simulink model "BANSHEE"  (Simulink 8.7)
settings: Solver=ode1  StartTime=0.0  StopTime=inf  FixedStep=Ts  MaxStep=1e-3  RelTol=1e-3
PostLoadFcn:
  | BANSHEE_init;
InitFcn:
  | BANSHEE_init;
values from neighbouring files (symbols this model uses):
  Ts = 100E-6    (= 0.0001)    [BANSHEE_init.m]
undefined symbols (not defined in the file or in its folder): Acid, Banshee_HWCtrl_IOs, Banshee_SEL751_Woodward_lib, DMS_slave_lib, DMSCommands, F1, F2, F3, fdesignblkfcn, Feeder1_lib, Feeder2_lib, Feeder3_lib, gcbh, generic_ethernet_cb, Lead, Left, relay_housing_lib, SM_UtilityService, SS_F1_RELAY_HOUSING, SS_F2_RELAY_HOUSING, SS_F3_RELAY_HOUSING, SS_Feeder1, SS_Feeder2, SS_Feeder3, SUBSTATION, TestSeq_slave_lib, TestSequenceCommands, type, utility_service_lib, V
libraries: powerlib x108, cables_lib x61, breaker_lib x53, rtio_generic_modbus x50, relay_modbus_lib x45, rtio_opalrt_op5142ex1 x37, transformer_lib x29, rteventslib x28, Load_lib x25, simulink x24, rtlab x20, ssn_lib x19
(part 7 of 9)

== system BANSHEE/SS_PV_BESS/EPC/LCL Filter 200kW1 ==
  note: High Resistor:
      | 10e6 ohms
      | Numerical Stability
  note: Create a three wire version that removes the Inv 4 port and 4 nuetral.
      | There is a reistor in parallel with the capacitor for the discharge voltage at shutoff.
  Bleed_R1 : powerlib/Elements/Series RLC Branch  LConnTagsString=__new0  RConnTagsString=__new0  BranchType=R  Resistance=filter_cap_bleed_res  Inductance=1e-3  SetiL0=off  InitialCurrent=0  Capacitance=filter_cap  Setx0=on  InitialVoltage=0  Measurements=None
  Bleed_R2 : powerlib/Elements/Series RLC Branch  LConnTagsString=__new0  RConnTagsString=__new0  BranchType=R  Resistance=filter_cap_bleed_res  Inductance=1e-3  SetiL0=off  InitialCurrent=0  Capacitance=filter_cap  Setx0=on  InitialVoltage=0  Measurements=None
  Bleed_R3 : powerlib/Elements/Series RLC Branch  LConnTagsString=__new0  RConnTagsString=__new0  BranchType=R  Resistance=filter_cap_bleed_res  Inductance=1e-3  SetiL0=off  InitialCurrent=0  Capacitance=filter_cap  Setx0=on  InitialVoltage=0  Measurements=None
  Capacitor_L1 : powerlib/Elements/Series RLC Branch  LConnTagsString=__new0  RConnTagsString=__new0  BranchType=RC  Resistance=filter_cap_res  Inductance=1e-3  SetiL0=off  InitialCurrent=0  Capacitance=filter_cap  Setx0=on  InitialVoltage=0  Measurements=None
  Capacitor_L2 : powerlib/Elements/Series RLC Branch  LConnTagsString=__new0  RConnTagsString=__new0  BranchType=RC  Resistance=filter_cap_res  Inductance=1e-3  SetiL0=off  InitialCurrent=0  Capacitance=filter_cap  Setx0=on  InitialVoltage=0  Measurements=None
  Capacitor_L3 : powerlib/Elements/Series RLC Branch  LConnTagsString=__new0  RConnTagsString=__new0  BranchType=RC  Resistance=filter_cap_res  Inductance=1e-3  SetiL0=off  InitialCurrent=0  Capacitance=filter_cap  Setx0=on  InitialVoltage=0  Measurements=None
  Inductor_Inv1 : powerlib/Elements/Series RLC Branch  LConnTagsString=__new0  RConnTagsString=__new0  BranchType=RL  Resistance=filter_inv_res  Inductance=filter_inv_ind  SetiL0=off  InitialCurrent=0  Capacitance=1e-6  Setx0=off  InitialVoltage=0  Measurements=None
  Inductor_Inv2 : powerlib/Elements/Series RLC Branch  LConnTagsString=__new0  RConnTagsString=__new0  BranchType=RL  Resistance=filter_inv_res  Inductance=filter_inv_ind  SetiL0=off  InitialCurrent=0  Capacitance=1e-6  Setx0=off  InitialVoltage=0  Measurements=None
  Inductor_Inv3 : powerlib/Elements/Series RLC Branch  LConnTagsString=__new0  RConnTagsString=__new0  BranchType=RL  Resistance=filter_inv_res  Inductance=filter_inv_ind  SetiL0=off  InitialCurrent=0  Capacitance=1e-6  Setx0=off  InitialVoltage=0  Measurements=None
  Inductor_Inv4 : powerlib/Elements/Series RLC Branch  LConnTagsString=__new0  RConnTagsString=__new0  BranchType=L  Resistance=1  Inductance=filter_inv_ind  SetiL0=off  InitialCurrent=0  Capacitance=1e-6  Setx0=off  InitialVoltage=0  Measurements=None
  Inductor_L1 : powerlib/Elements/Series RLC Branch  LConnTagsString=__new0  RConnTagsString=__new0  BranchType=RL  Resistance=filter_line_res  Inductance=filter_line_ind  SetiL0=off  InitialCurrent=0  Capacitance=1e-6  Setx0=off  InitialVoltage=0  Measurements=None
  Inductor_L2 : powerlib/Elements/Series RLC Branch  LConnTagsString=__new0  RConnTagsString=__new0  BranchType=RL  Resistance=filter_line_res  Inductance=filter_line_ind  SetiL0=off  InitialCurrent=0  Capacitance=1e-6  Setx0=off  InitialVoltage=0  Measurements=None
  Inductor_L3 : powerlib/Elements/Series RLC Branch  LConnTagsString=__new0  RConnTagsString=__new0  BranchType=RL  Resistance=filter_line_res  Inductance=filter_line_ind  SetiL0=off  InitialCurrent=0  Capacitance=1e-6  Setx0=off  InitialVoltage=0  Measurements=None
  Three-Phase Series RLC Branch : powerlib/Elements/Three-Phase Series RLC Branch  LConnTagsString=A|B|C  RConnTagsString=A|B|C  BranchType=R  Resistance=1e6  Inductance=1e-3  Capacitance=1e-6  Measurements=None
  A : PMIOPort  Port=1  Side=Left
  B : PMIOPort  Port=2  Side=Left
  C : PMIOPort  Port=3  Side=Left
  N : PMIOPort  Port=4  Side=Left
  Inv_1 : PMIOPort  Port=5  Side=Right  mask{filter_line_ind=[], filter_cap=0, filter_inv_ind=0}
      mask prompts: filter_line_ind "Line Filter Inductor (H)"; filter_cap "Filter Capacitor (F)"; filter_inv_ind "Inverter Filter Inductor (H)"
  Inv_2 : PMIOPort  Port=6  Side=Right
  Inv_3 : PMIOPort  Port=7  Side=Right
  Inv_4 : PMIOPort  Port=8  Side=Right
  connections:
  Inductor_L1/RConn1 -- Inductor_Inv1/LConn1 -- Capacitor_L1/LConn1 -- Bleed_R1/LConn1
  Inv_1/RConn1 -- Inductor_Inv1/RConn1
  A/RConn1 -- Inductor_L1/LConn1
  Inductor_L2/RConn1 -- Inductor_Inv2/LConn1 -- Capacitor_L2/LConn1 -- Bleed_R2/LConn1
  Inv_2/RConn1 -- Inductor_Inv2/RConn1
  B/RConn1 -- Inductor_L2/LConn1
  Inductor_L3/RConn1 -- Inductor_Inv3/LConn1 -- Capacitor_L3/LConn1 -- Bleed_R3/LConn1
  Inv_3/RConn1 -- Inductor_Inv3/RConn1
  C/RConn1 -- Inductor_L3/LConn1
  N/RConn1 -- Capacitor_L1/RConn1 -- Bleed_R1/RConn1 -- Capacitor_L2/RConn1 -- Bleed_R2/RConn1 -- Capacitor_L3/RConn1 -- Bleed_R3/RConn1 -- Inductor_Inv4/LConn1
  Inv_4/RConn1 -- Inductor_Inv4/RConn1

== system BANSHEE/SS_PV_BESS/EPC/LCL Filter 200kW2 ==
  note: High Resistor:
      | 10e6 ohms
      | Numerical Stability
  note: Create a three wire version that removes the Inv 4 port and 4 nuetral.
      | There is a reistor in parallel with the capacitor for the discharge voltage at shutoff.
  Bleed_R1 : powerlib/Elements/Series RLC Branch  LConnTagsString=__new0  RConnTagsString=__new0  BranchType=R  Resistance=filter_cap_bleed_res  Inductance=1e-3  SetiL0=off  InitialCurrent=0  Capacitance=filter_cap  Setx0=on  InitialVoltage=0  Measurements=None
  Bleed_R2 : powerlib/Elements/Series RLC Branch  LConnTagsString=__new0  RConnTagsString=__new0  BranchType=R  Resistance=filter_cap_bleed_res  Inductance=1e-3  SetiL0=off  InitialCurrent=0  Capacitance=filter_cap  Setx0=on  InitialVoltage=0  Measurements=None
  Bleed_R3 : powerlib/Elements/Series RLC Branch  LConnTagsString=__new0  RConnTagsString=__new0  BranchType=R  Resistance=filter_cap_bleed_res  Inductance=1e-3  SetiL0=off  InitialCurrent=0  Capacitance=filter_cap  Setx0=on  InitialVoltage=0  Measurements=None
  Capacitor_L1 : powerlib/Elements/Series RLC Branch  LConnTagsString=__new0  RConnTagsString=__new0  BranchType=RC  Resistance=filter_cap_res  Inductance=1e-3  SetiL0=off  InitialCurrent=0  Capacitance=filter_cap  Setx0=on  InitialVoltage=0  Measurements=None
  Capacitor_L2 : powerlib/Elements/Series RLC Branch  LConnTagsString=__new0  RConnTagsString=__new0  BranchType=RC  Resistance=filter_cap_res  Inductance=1e-3  SetiL0=off  InitialCurrent=0  Capacitance=filter_cap  Setx0=on  InitialVoltage=0  Measurements=None
  Capacitor_L3 : powerlib/Elements/Series RLC Branch  LConnTagsString=__new0  RConnTagsString=__new0  BranchType=RC  Resistance=filter_cap_res  Inductance=1e-3  SetiL0=off  InitialCurrent=0  Capacitance=filter_cap  Setx0=on  InitialVoltage=0  Measurements=None
  Inductor_Inv1 : powerlib/Elements/Series RLC Branch  LConnTagsString=__new0  RConnTagsString=__new0  BranchType=RL  Resistance=filter_inv_res  Inductance=filter_inv_ind  SetiL0=off  InitialCurrent=0  Capacitance=1e-6  Setx0=off  InitialVoltage=0  Measurements=None
  Inductor_Inv2 : powerlib/Elements/Series RLC Branch  LConnTagsString=__new0  RConnTagsString=__new0  BranchType=RL  Resistance=filter_inv_res  Inductance=filter_inv_ind  SetiL0=off  InitialCurrent=0  Capacitance=1e-6  Setx0=off  InitialVoltage=0  Measurements=None
  Inductor_Inv3 : powerlib/Elements/Series RLC Branch  LConnTagsString=__new0  RConnTagsString=__new0  BranchType=RL  Resistance=filter_inv_res  Inductance=filter_inv_ind  SetiL0=off  InitialCurrent=0  Capacitance=1e-6  Setx0=off  InitialVoltage=0  Measurements=None
  Inductor_Inv4 : powerlib/Elements/Series RLC Branch  LConnTagsString=__new0  RConnTagsString=__new0  BranchType=L  Resistance=1  Inductance=filter_inv_ind  SetiL0=off  InitialCurrent=0  Capacitance=1e-6  Setx0=off  InitialVoltage=0  Measurements=None
  Inductor_L1 : powerlib/Elements/Series RLC Branch  LConnTagsString=__new0  RConnTagsString=__new0  BranchType=RL  Resistance=filter_line_res  Inductance=filter_line_ind  SetiL0=off  InitialCurrent=0  Capacitance=1e-6  Setx0=off  InitialVoltage=0  Measurements=None
  Inductor_L2 : powerlib/Elements/Series RLC Branch  LConnTagsString=__new0  RConnTagsString=__new0  BranchType=RL  Resistance=filter_line_res  Inductance=filter_line_ind  SetiL0=off  InitialCurrent=0  Capacitance=1e-6  Setx0=off  InitialVoltage=0  Measurements=None
  Inductor_L3 : powerlib/Elements/Series RLC Branch  LConnTagsString=__new0  RConnTagsString=__new0  BranchType=RL  Resistance=filter_line_res  Inductance=filter_line_ind  SetiL0=off  InitialCurrent=0  Capacitance=1e-6  Setx0=off  InitialVoltage=0  Measurements=None
  Three-Phase Series RLC Branch : powerlib/Elements/Three-Phase Series RLC Branch  LConnTagsString=A|B|C  RConnTagsString=A|B|C  BranchType=R  Resistance=1e6  Inductance=1e-3  Capacitance=1e-6  Measurements=None
  A : PMIOPort  Port=1  Side=Left
  B : PMIOPort  Port=2  Side=Left
  C : PMIOPort  Port=3  Side=Left
  N : PMIOPort  Port=4  Side=Left
  Inv_1 : PMIOPort  Port=5  Side=Right  mask{filter_line_ind=[], filter_cap=0, filter_inv_ind=0}
      mask prompts: filter_line_ind "Line Filter Inductor (H)"; filter_cap "Filter Capacitor (F)"; filter_inv_ind "Inverter Filter Inductor (H)"
  Inv_2 : PMIOPort  Port=6  Side=Right
  Inv_3 : PMIOPort  Port=7  Side=Right
  Inv_4 : PMIOPort  Port=8  Side=Right
  connections:
  Inductor_L1/RConn1 -- Inductor_Inv1/LConn1 -- Capacitor_L1/LConn1 -- Bleed_R1/LConn1
  Inv_1/RConn1 -- Inductor_Inv1/RConn1
  A/RConn1 -- Inductor_L1/LConn1
  Inductor_L2/RConn1 -- Inductor_Inv2/LConn1 -- Capacitor_L2/LConn1 -- Bleed_R2/LConn1
  Inv_2/RConn1 -- Inductor_Inv2/RConn1
  B/RConn1 -- Inductor_L2/LConn1
  Inductor_L3/RConn1 -- Inductor_Inv3/LConn1 -- Capacitor_L3/LConn1 -- Bleed_R3/LConn1
  Inv_3/RConn1 -- Inductor_Inv3/RConn1
  C/RConn1 -- Inductor_L3/LConn1
  N/RConn1 -- Capacitor_L1/RConn1 -- Bleed_R1/RConn1 -- Capacitor_L2/RConn1 -- Bleed_R2/RConn1 -- Capacitor_L3/RConn1 -- Bleed_R3/RConn1 -- Inductor_Inv4/LConn1
  Inv_4/RConn1 -- Inductor_Inv4/RConn1

== system BANSHEE/SC_ctrl/EPC Inverter/16TSDIn/16 TSDOut GR3/Din/Dout ch16-23 ==
  Bus Creator3 : BusCreator  Inputs=8
  times17 : Constant  Value=[0.05 0.15 0.25 0.35]
  times18 : Constant  Value=[0.1 0.2 0.3 0.4]
  times19 : Constant  Value=[0.15 0.25 0.35 0.45]
  times20 : Constant  Value=[0.2 0.3 0.4 0.5]
  times21 : Constant  Value=[0.25 0.35 0.45 0.55]
  times22 : Constant  Value=[0.3 0.4 0.5 0.6]
  times23 : Constant  Value=[0.3 0.4 0.5 0.6]
  times24 : Constant  Value=[0 0.1 0.2 0.3]
  Out1 : Outport
  wires:
  times24/1 -> Bus Creator3/1  "times17"
  times17/1 -> Bus Creator3/2  "times18"
  times18/1 -> Bus Creator3/3  "times19"
  times19/1 -> Bus Creator3/4  "times20"
  times20/1 -> Bus Creator3/5  "times21"
  times21/1 -> Bus Creator3/6  "times22"
  times22/1 -> Bus Creator3/7  "times23"
  times23/1 -> Bus Creator3/8  "times24"
  Bus Creator3/1 -> Out1/1

== system BANSHEE/SC_ctrl/EPC Inverter/16TSDIn/16 TSDOut GR3/Din/Dout ch24-31 ==
  Bus Creator4 : BusCreator  Inputs=8
  times25 : Constant  Value=[0.05 0.15 0.25 0.35]
  times26 : Constant  Value=[0.1 0.2 0.3 0.4]
  times27 : Constant  Value=[0.15 0.25 0.35 0.45]
  times28 : Constant  Value=[0.2 0.3 0.4 0.5]
  times29 : Constant  Value=[0.25 0.35 0.45 0.55]
  times30 : Constant  Value=[0.3 0.4 0.5 0.6]
  times31 : Constant  Value=[0.3 0.4 0.5 0.6]
  times32 : Constant  Value=[0 0.1 0.2 0.3]
  Out1 : Outport
  wires:
  times32/1 -> Bus Creator4/1  "times25"
  times25/1 -> Bus Creator4/2  "times26"
  times26/1 -> Bus Creator4/3  "times27"
  times27/1 -> Bus Creator4/4  "times28"
  times28/1 -> Bus Creator4/5  "times29"
  times29/1 -> Bus Creator4/6  "times30"
  times30/1 -> Bus Creator4/7  "times31"
  times31/1 -> Bus Creator4/8  "times32"
  Bus Creator4/1 -> Out1/1

== system BANSHEE/SC_ctrl/EPC Inverter/16TSDIn/16 TSDOut GR3/Dout state ctrl ==
  Bus Creator : BusCreator  Inputs=2
  Dout_CH16_CH23 : Subsystem
  Dout_CH24_CH31 : Subsystem
  Event State OUT : Outport
  wires:
  Bus Creator/1 -> Event State OUT/1
  Dout_CH16_CH23/1(Dout_CH8_CH15) -> Bus Creator/1  "CH16-23"
  Dout_CH24_CH31/1(Dout_CH8_CH15) -> Bus Creator/2  "CH24-31"

== system BANSHEE/SM_UtilityService/Banshee_HWCtrl_IOs/SEL751_DigitalAnalog_IO_OpBlocks/F1 ==
  Substation : Inport
  Feeder : Inport  Port=2
  DTT : Inport  Port=3
  TS_SQ : Inport  Port=4
  Logical Operator : Logic  AllPortsSameDT=off  OutDataTypeStr=boolean
  Logical Operator1 : Logic  Operator=OR  Inputs=3  AllPortsSameDT=off  OutDataTypeStr=boolean
  Logical Operator2 : Logic  Operator=OR  AllPortsSameDT=off  OutDataTypeStr=boolean
  Logical Operator3 : Logic  Operator=NOT  AllPortsSameDT=off  OutDataTypeStr=boolean
  Logical Operator5 : Logic  Operator=NOT  AllPortsSameDT=off  OutDataTypeStr=boolean
  trip : Outport
  wires:
  DTT/1 -> Logical Operator2/1
  Feeder/1 -> Logical Operator5/1
  Logical Operator5/1 -> Logical Operator1/2
  Substation/1 -> Logical Operator3/1
  Logical Operator3/1 -> Logical Operator1/1
  Logical Operator1/1 -> Logical Operator/1
  Logical Operator/1 -> trip/1
  Logical Operator2/1 -> Logical Operator/2
  TS_SQ/1 -> Logical Operator1/3, Logical Operator2/2

== system BANSHEE/SM_UtilityService/Banshee_HWCtrl_IOs/SEL751_DigitalAnalog_IO_OpBlocks/F2 ==
  Substation : Inport
  Feeder : Inport  Port=2
  DTT : Inport  Port=3
  TS_SQ : Inport  Port=4
  Logical Operator : Logic  AllPortsSameDT=off  OutDataTypeStr=boolean
  Logical Operator1 : Logic  Operator=OR  Inputs=3  AllPortsSameDT=off  OutDataTypeStr=boolean
  Logical Operator2 : Logic  Operator=OR  AllPortsSameDT=off  OutDataTypeStr=boolean
  Logical Operator3 : Logic  Operator=NOT  AllPortsSameDT=off  OutDataTypeStr=boolean
  Logical Operator5 : Logic  Operator=NOT  AllPortsSameDT=off  OutDataTypeStr=boolean
  trip : Outport
  wires:
  DTT/1 -> Logical Operator2/1
  Feeder/1 -> Logical Operator5/1
  Logical Operator5/1 -> Logical Operator1/2
  Substation/1 -> Logical Operator3/1
  Logical Operator3/1 -> Logical Operator1/1
  Logical Operator1/1 -> Logical Operator/1
  Logical Operator/1 -> trip/1
  Logical Operator2/1 -> Logical Operator/2
  TS_SQ/1 -> Logical Operator1/3, Logical Operator2/2

== system BANSHEE/SM_UtilityService/Banshee_HWCtrl_IOs/SEL751_DigitalAnalog_IO_OpBlocks/F3 ==
  Substation : Inport
  Feeder : Inport  Port=2
  DTT : Inport  Port=3
  TS_SQ : Inport  Port=4
  Logical Operator : Logic  AllPortsSameDT=off  OutDataTypeStr=boolean
  Logical Operator1 : Logic  Operator=OR  Inputs=3  AllPortsSameDT=off  OutDataTypeStr=boolean
  Logical Operator2 : Logic  Operator=OR  AllPortsSameDT=off  OutDataTypeStr=boolean
  Logical Operator3 : Logic  Operator=NOT  AllPortsSameDT=off  OutDataTypeStr=boolean
  Logical Operator5 : Logic  Operator=NOT  AllPortsSameDT=off  OutDataTypeStr=boolean
  trip : Outport
  wires:
  DTT/1 -> Logical Operator2/1
  Feeder/1 -> Logical Operator5/1
  Logical Operator5/1 -> Logical Operator1/2
  Substation/1 -> Logical Operator3/1
  Logical Operator3/1 -> Logical Operator1/1
  Logical Operator1/1 -> Logical Operator/1
  Logical Operator/1 -> trip/1
  Logical Operator2/1 -> Logical Operator/2
  TS_SQ/1 -> Logical Operator1/3, Logical Operator2/2

== system BANSHEE/SM_UtilityService/Banshee_HWCtrl_IOs/Woodward Outputs - Diesel - Gen2/DIO - Gr3 ==
  Dout : Inport
  Bus Creator : BusCreator  Inputs=1
  Bus Selector1 : BusSelector  OutputSignals=DI_CH08-15  OutputAsBus=on
  Conditioning1 : Subsystem
  DigitalIn1 : rtio_opalrt_common/DigitalIn  CtrlName='OpCtrl'  portNb=6  FcnNos=Slot 3 Module A Subsection 2  size=1  maxcount=8  count=8  sampleTime=0  numchan=8
      settings: AttributesFormatString=%<CtrlName>
  DigitalOut1 : rtio_opalrt_common/DigitalOut  CtrlName='OpCtrl'  portNb=6  FcnNos=Slot 3 Module B Subsection 2  size=1  maxcount=8  count=8  numchan=8
      settings: AttributesFormatString=%<CtrlName>
  Terminator1 : Terminator
  Terminator6 : Terminator
  DIn : Outport
  wires:
  DigitalOut1/1 -> Terminator1/1
  Dout/1 -> Bus Selector1/1
  Bus Selector1/1 -> DigitalOut1/1
  DigitalIn1/2 -> Terminator6/1
  DigitalIn1/1 -> Conditioning1/1(In1)  "DI_CH08-15"
  Bus Creator/1 -> DIn/1
  Conditioning1/1(Out1) -> Bus Creator/1

== system BANSHEE/SM_UtilityService/Banshee_HWCtrl_IOs/Woodward Outputs - Diesel - Gen2/DIO - Woodward ==
  note: Copyright (c) 2016 Massachusetts Institute of Technology
      | Permission is hereby granted, free of charge, to any person obtaining a copy of this software and associated documentation files (the "Software"), to deal
      | in the Software without restriction, including without limitation the rights to use, copy, modify, merge, publish, distribute, sublicense, and/or sell copies of the
      | Software, and to permit persons to whom the Software is furnished to do so, subject to the following conditions:
      |
      | THE SOFTWARE IS PROVIDED "AS IS", WITHOUT WARRANTY OF ANY KIND, EXPRESS OR IMPLIED, INCLUDING BUT NOT LIMITED TO THE
      | WARRANTIES OF MERCHANTABILITY, FITNESS FOR A PARTICULAR PURPOSE AND NONINFRINGEMENT. IN NO EVENT SHALL THE AUTHORS
      | OR COPYRIGHT HOLDERS BE LIABLE FOR ANY CLAIM, DAMAGES OR OTHER LIABILITY, WHETHER IN AN ACTION OF CONTRACT, TORT OR
      | OTHERWISE, ARISING FROM, OUT OF OR IN CONNECTION WITH THE SOFTWARE OR THE USE OR OTHER DEALINGS IN THE SOFTWARE
  note: Ch08-11
  note: These are the inputs to
      | the HIL Outputs.
  Din_Wood : Inport
  Gen2 MCB Status : Inport  Port=2
  Add2 : Sum
  Add3 : Sum
  Bus Creator : BusCreator  Inputs=1
  Bus Selector5 : BusSelector  OutputSignals=DI_CH08-15.Gen2_Starter,DI_CH08-15.Gen2_Fuel
  Bus Selector6 : BusSelector  OutputSignals=DI_CH08-15.Gen2_Open_GCB,DI_CH08-15.Gen2_Close_GCB,DI_CH08-15.Gen2_Open_MCB,DI_CH08-15.Gen2_Close_MCB
  Compare To Zero{7..8,10..12} (5 alike) : simulink/Logic and Bit Operations/Compare To Zero  relop=>  OutDataTypeStr=boolean
  Compare To Zero13 : simulink/Logic and Bit Operations/Compare To Zero  relop=<=  OutDataTypeStr=boolean
  Constant : Constant  Value=0
  Constant1 : Constant
  Constant3 : Constant
  Constant4 : Constant
  Constant5 : Constant  Value=0
  Data Type Conversion{,1..3} (4 alike) : DataTypeConversion  OutDataTypeStr=double
  Logical Operator1 : Logic  Operator=NOT  AllPortsSameDT=off  OutDataTypeStr=boolean
  Mux1 : Mux  Inputs=8
  S-R Flip-Flop3 : simulink_extras/Flip Flops/S-R Flip-Flop  initial_condition=1
  S-R Flip-Flop4 : simulink_extras/Flip Flops/S-R Flip-Flop  initial_condition=1
  S-R Flip-Flop5 : simulink_extras/Flip Flops/S-R Flip-Flop  initial_condition=0
  Switch5 : Switch  Threshold=0.5
  Terminator : Terminator
  Terminator1 : Terminator
  DIn1 : Outport
  Gen2 Fuel Enable : Outport  Port=2
  Gen2 GCB : Outport  Port=3
  Gen2 MCB : Outport  Port=4
  wires:
  Constant1/1 -> Mux1/1  "Estop"
  Data Type Conversion3/1 -> Mux1/8
  Data Type Conversion2/1 -> Mux1/7
  Data Type Conversion1/1 -> Mux1/6
  Constant/1 -> Mux1/4, Mux1/3, Mux1/2
  S-R Flip-Flop5/2 -> Terminator1/1
  S-R Flip-Flop4/2 -> Terminator/1
  Din_Wood/1 -> Bus Selector5/1, Bus Selector6/1
  Bus Creator/1 -> DIn1/1
  Mux1/1 -> Bus Creator/1  "DI_CH08-15"
  S-R Flip-Flop3/1 -> Data Type Conversion1/1, Add2/1
  Bus Selector6/1 -> Compare To Zero7/1  "<Gen2_Open_GCB>"
  Compare To Zero7/1 -> S-R Flip-Flop3/1
  Compare To Zero8/1 -> S-R Flip-Flop3/2
  Bus Selector6/4 -> Compare To Zero11/1  "<Gen2_Close_MCB>"
  Compare To Zero11/1 -> S-R Flip-Flop4/2
  Bus Selector6/3 -> Compare To Zero10/1  "<Gen2_Open_MCB>"
  Compare To Zero10/1 -> S-R Flip-Flop4/1
  Bus Selector6/2 -> Compare To Zero8/1  "<Gen2_Close_GCB>"
  S-R Flip-Flop4/1 -> Add3/2
  Add2/1 -> Gen2 GCB/1
  Add3/1 -> Gen2 MCB/1
  Constant3/1 -> Add2/2, Add3/1
  Bus Selector5/1 -> Compare To Zero12/1  "<Gen2_Starter>"
  Bus Selector5/2 -> Compare To Zero13/1  "<Gen2_Fuel>"
  S-R Flip-Flop5/1 -> Switch5/2
  Compare To Zero12/1 -> S-R Flip-Flop5/1
  Constant5/1 -> Switch5/3
  Constant4/1 -> Switch5/1
  Compare To Zero13/1 -> S-R Flip-Flop5/2
  Switch5/1 -> Gen2 Fuel Enable/1
  Gen2 MCB Status/1 -> Logical Operator1/1, Data Type Conversion2/1
  S-R Flip-Flop3/2 -> Data Type Conversion3/1
  Logical Operator1/1 -> Data Type Conversion/1
  Data Type Conversion/1 -> Mux1/5

== system BANSHEE/SM_UtilityService/Banshee_HWCtrl_IOs/Woodward Outputs - Diesel - Gen2/DOUT type config ==
  note: The Constants are used to select Digital Output type:
      | - 0: Time-Stamped Digital Output
      | - 1: Pulse-Width Modulated DIgital Output
  DataIn Send1 : rtio_opalrt_common/DataIn Send  CtrlName='OpCtrl'  FcnNos=12  width=1  portType=double  checkVersion=off  expectedId=0  expectedVersion=0  opComp=>=
      settings: AttributesFormatString=%<CtrlName>
  Subsection 4 DOUT type : Constant
  Terminator1 : Terminator
  wires:
  Subsection 4 DOUT type/1 -> DataIn Send1/1
  DataIn Send1/1 -> Terminator1/1

== system BANSHEE/SM_UtilityService/Banshee_HWCtrl_IOs/Woodward Outputs - Diesel - Gen2/Woodward Primary Inputs - Gen2 ==
  note: Copyright (c) 2016 Massachusetts Institute of Technology
      | Permission is hereby granted, free of charge, to any person obtaining a copy of this software and associated documentation files (the "Software"), to deal
      | in the Software without restriction, including without limitation the rights to use, copy, modify, merge, publish, distribute, sublicense, and/or sell copies of the
      | Software, and to permit persons to whom the Software is furnished to do so, subject to the following conditions:
      |
      | THE SOFTWARE IS PROVIDED "AS IS", WITHOUT WARRANTY OF ANY KIND, EXPRESS OR IMPLIED, INCLUDING BUT NOT LIMITED TO THE
      | WARRANTIES OF MERCHANTABILITY, FITNESS FOR A PARTICULAR PURPOSE AND NONINFRINGEMENT. IN NO EVENT SHALL THE AUTHORS
      | OR COPYRIGHT HOLDERS BE LIABLE FOR ANY CLAIM, DAMAGES OR OTHER LIABILITY, WHETHER IN AN ACTION OF CONTRACT, TORT OR
      | OTHERWISE, ARISING FROM, OUT OF OR IN CONNECTION WITH THE SOFTWARE OR THE USE OR OTHER DEALINGS IN THE SOFTWARE
  note: Diesel -> Gen2
  WoodwardBias : Inport
  Bus Creator1 : BusCreator  Inputs=4
  Bus Selector5 : BusSelector  OutputSignals=gen2_GOV_bias,gen2_AVR_bias
  Constant8 : Constant  Value=0
  Constant9 : Constant  Value=0
  Divide2 : Product  Inputs=*/
  Divide3 : Product  Inputs=*/
  Gen2 Ref AVR : Constant  Value=1.00
  Gen2 Ref GOV : Constant  Value=1.00
  Lowpass Filter2 : Subsystem  DialogController=fdesignblkfcn  DialogControllerArgs=DataTag2  InitFcn=fdesignblkfcn(gcbh, {'InitFcn'});  mask(Lowpass Filter){}
      mask help: Design a lowpass filter
      settings: CopyFcn=fdesignblkfcn(gcbh, {'CopyFcn'});
      mask Help: helpview(mapfilelocation('dsp'), 'dsplowpassfilter');
      mask Display: disp('Lowpass')
  Lowpass Filter3 : Subsystem  DialogController=fdesignblkfcn  DialogControllerArgs=DataTag4  InitFcn=fdesignblkfcn(gcbh, {'InitFcn'});  mask(Lowpass Filter){}
      mask help: Design a lowpass filter
      settings: CopyFcn=fdesignblkfcn(gcbh, {'CopyFcn'});
      mask Help: helpview(mapfilelocation('dsp'), 'dsplowpassfilter');
      mask Display: disp('Lowpass')
  ScalingBias : Constant  Value=20
  SimulatedBiasValues : Constant  Value=0
  Sum2 : Sum  Inputs=|+-
  Sum3 : Sum  Inputs=|+-
  Switch2 : Switch  Threshold=0.5
  Switch3 : Switch  Threshold=0.5
  bias_enable_for_woodward_ctrl : Constant
  Gen2 Gov and AVR : Outport
  wires:
  bias_enable_for_woodward_ctrl/1 -> Switch2/2, Switch3/2
  ScalingBias/1 -> Divide2/2, Divide3/2
  Divide2/1 -> Sum2/1
  Divide3/1 -> Sum3/1
  Constant8/1 -> Sum2/2
  Constant9/1 -> Sum3/2
  Sum2/1 -> Lowpass Filter2/1(In)
  Switch2/1 -> Bus Creator1/3  "Gen2 GOV"
  Switch3/1 -> Bus Creator1/4  "Gen2 AVR"
  Sum3/1 -> Lowpass Filter3/1(In)
  SimulatedBiasValues/1 -> Switch2/3, Switch3/3
  Lowpass Filter2/1(Out) -> Switch2/1
  Lowpass Filter3/1(Out) -> Switch3/1
  Gen2 Ref AVR/1 -> Bus Creator1/2  "Gen2 Ref AVR"
  Gen2 Ref GOV/1 -> Bus Creator1/1  "Gen2 Ref GOV"
  Bus Creator1/1 -> Gen2 Gov and AVR/1
  WoodwardBias/1 -> Bus Selector5/1
  Bus Selector5/1 -> Divide2/1  "<gen2_GOV_bias>"
  Bus Selector5/2 -> Divide3/1  "<gen2_AVR_bias>"

== system BANSHEE/SM_UtilityService/Banshee_HWCtrl_IOs/Woodward Outputs - NGCHP - Gen1/DIO - Gr3 ==
  Dout : Inport
  Bus Creator : BusCreator  Inputs=1
  Bus Selector : BusSelector  OutputSignals=DI_CH00-07  OutputAsBus=on
  Conditioning : Subsystem
  DigitalIn : rtio_opalrt_common/DigitalIn  CtrlName='OpCtrl'  portNb=5  FcnNos=Slot 3 Module A Subsection 1  size=1  maxcount=8  count=8  sampleTime=0  numchan=8
      settings: AttributesFormatString=%<CtrlName>
  DigitalOut : rtio_opalrt_common/DigitalOut  CtrlName='OpCtrl'  portNb=5  FcnNos=Slot 3 Module B Subsection 1  size=1  maxcount=8  count=8  numchan=8
      settings: AttributesFormatString=%<CtrlName>
  Terminator3 : Terminator
  Terminator5 : Terminator
  DIn : Outport
  wires:
  DigitalOut/1 -> Terminator3/1
  Dout/1 -> Bus Selector/1
  Bus Selector/1 -> DigitalOut/1
  DigitalIn/2 -> Terminator5/1
  DigitalIn/1 -> Conditioning/1(In1)  "DI_CH00-07"
  Bus Creator/1 -> DIn/1
  Conditioning/1(Out1) -> Bus Creator/1

== system BANSHEE/SM_UtilityService/Banshee_HWCtrl_IOs/Woodward Outputs - NGCHP - Gen1/DIO - Woodward ==
  note: These are the inputs to
      | the HIL Outputs.
  note: Ch00-03
  note: Copyright (c) 2016 Massachusetts Institute of Technology
      | Permission is hereby granted, free of charge, to any person obtaining a copy of this software and associated documentation files (the "Software"), to deal
      | in the Software without restriction, including without limitation the rights to use, copy, modify, merge, publish, distribute, sublicense, and/or sell copies of the
      | Software, and to permit persons to whom the Software is furnished to do so, subject to the following conditions:
      |
      | THE SOFTWARE IS PROVIDED "AS IS", WITHOUT WARRANTY OF ANY KIND, EXPRESS OR IMPLIED, INCLUDING BUT NOT LIMITED TO THE
      | WARRANTIES OF MERCHANTABILITY, FITNESS FOR A PARTICULAR PURPOSE AND NONINFRINGEMENT. IN NO EVENT SHALL THE AUTHORS
      | OR COPYRIGHT HOLDERS BE LIABLE FOR ANY CLAIM, DAMAGES OR OTHER LIABILITY, WHETHER IN AN ACTION OF CONTRACT, TORT OR
      | OTHERWISE, ARISING FROM, OUT OF OR IN CONNECTION WITH THE SOFTWARE OR THE USE OR OTHER DEALINGS IN THE SOFTWARE
  Din_Wood : Inport
  Gen1 MCB Status : Inport  Port=2
  Add : Sum
  Add1 : Sum
  Bus Creator : BusCreator  Inputs=1
  Bus Selector : BusSelector  OutputSignals=DI_CH00-07.Gen1_Starter,DI_CH00-07.Gen1_Fuel
  Bus Selector3 : BusSelector  OutputSignals=DI_CH00-07.Gen1_Open_GCB,DI_CH00-07.Gen1_Close_GCB,DI_CH00-07.Gen1_Open_MCB,DI_CH00-07.Gen1_Close_MCB
  Compare To Zero{,1,3..4} (4 alike) : simulink/Logic and Bit Operations/Compare To Zero  relop=>  OutDataTypeStr=boolean
  Constant : Constant
  Constant1 : Constant
  Constant3 : Constant  Value=0
  Data Type Conversion{,1..3} (4 alike) : DataTypeConversion  OutDataTypeStr=double
  Data Type Conversion4 : DataTypeConversion
  Logical Operator : Logic  Operator=NOT  AllPortsSameDT=off  OutDataTypeStr=boolean
  Logical Operator2 : Logic  Operator=NOR  AllPortsSameDT=off  OutDataTypeStr=boolean
  Mux2 : Mux  Inputs=8
  S-R Flip-Flop : simulink_extras/Flip Flops/S-R Flip-Flop  initial_condition=1
  S-R Flip-Flop1 : simulink_extras/Flip Flops/S-R Flip-Flop  initial_condition=1
  Terminator : Terminator
  Gen1 Fuel Enable : Outport
  Gen1 GCB : Outport  Port=2
  Gen1 MCB : Outport  Port=3
  DIn1 : Outport  Port=4
  wires:
  Constant1/1 -> Mux2/1  "Estop"
  Data Type Conversion4/1 -> Gen1 Fuel Enable/1
  Bus Selector3/2 -> Compare To Zero1/1  "<Gen1_Close_GCB>"
  Bus Selector3/1 -> Compare To Zero/1  "<Gen1_Open_GCB>"
  Din_Wood/1 -> Bus Selector3/1, Bus Selector/1
  Bus Creator/1 -> DIn1/1
  S-R Flip-Flop/1 -> Add/1, Data Type Conversion2/1
  Compare To Zero/1 -> S-R Flip-Flop/1
  Compare To Zero1/1 -> S-R Flip-Flop/2
  Bus Selector3/4 -> Compare To Zero4/1  "<Gen1_Close_MCB>"
  Compare To Zero4/1 -> S-R Flip-Flop1/2
  Compare To Zero3/1 -> S-R Flip-Flop1/1
  S-R Flip-Flop1/1 -> Add1/2
  Add/1 -> Gen1 GCB/1
  Add1/1 -> Gen1 MCB/1
  Constant/1 -> Add/2, Add1/1
  Bus Selector/1 -> Logical Operator2/1  "<Gen1_Starter>"
  Bus Selector/2 -> Logical Operator2/2  "<Gen1_Fuel>"
  Bus Selector3/3 -> Compare To Zero3/1  "<Gen1_Open_MCB>"
  Gen1 MCB Status/1 -> Data Type Conversion1/1, Logical Operator/1
  S-R Flip-Flop/2 -> Data Type Conversion3/1
  Data Type Conversion/1 -> Mux2/5
  Logical Operator/1 -> Data Type Conversion/1
  Logical Operator2/1 -> Data Type Conversion4/1
  Constant3/1 -> Mux2/4, Mux2/3, Mux2/2
  Mux2/1 -> Bus Creator/1  "DI_CH00-07"
  Data Type Conversion3/1 -> Mux2/8
  Data Type Conversion1/1 -> Mux2/7
  Data Type Conversion2/1 -> Mux2/6
  S-R Flip-Flop1/2 -> Terminator/1

== system BANSHEE/SM_UtilityService/Banshee_HWCtrl_IOs/Woodward Outputs - NGCHP - Gen1/DOUT type config ==
  note: The Constants are used to select Digital Output type:
      | - 0: Time-Stamped Digital Output
      | - 1: Pulse-Width Modulated DIgital Output
  DataIn Send : rtio_opalrt_common/DataIn Send  CtrlName='OpCtrl'  FcnNos=11  width=1  portType=double  checkVersion=off  expectedId=0  expectedVersion=0  opComp=>=
      settings: AttributesFormatString=%<CtrlName>
  Subsection 3 DOUT type : Constant
  Terminator2 : Terminator
  wires:
  Subsection 3 DOUT type/1 -> DataIn Send/1
  DataIn Send/1 -> Terminator2/1

== system BANSHEE/SM_UtilityService/Banshee_HWCtrl_IOs/Woodward Outputs - NGCHP - Gen1/Woodward Primary Inputs - Gen1 ==
  note: NG-CHP -> Gen1
  note: Copyright (c) 2016 Massachusetts Institute of Technology
      | Permission is hereby granted, free of charge, to any person obtaining a copy of this software and associated documentation files (the "Software"), to deal
      | in the Software without restriction, including without limitation the rights to use, copy, modify, merge, publish, distribute, sublicense, and/or sell copies of the
      | Software, and to permit persons to whom the Software is furnished to do so, subject to the following conditions:
      |
      | THE SOFTWARE IS PROVIDED "AS IS", WITHOUT WARRANTY OF ANY KIND, EXPRESS OR IMPLIED, INCLUDING BUT NOT LIMITED TO THE
      | WARRANTIES OF MERCHANTABILITY, FITNESS FOR A PARTICULAR PURPOSE AND NONINFRINGEMENT. IN NO EVENT SHALL THE AUTHORS
      | OR COPYRIGHT HOLDERS BE LIABLE FOR ANY CLAIM, DAMAGES OR OTHER LIABILITY, WHETHER IN AN ACTION OF CONTRACT, TORT OR
      | OTHERWISE, ARISING FROM, OUT OF OR IN CONNECTION WITH THE SOFTWARE OR THE USE OR OTHER DEALINGS IN THE SOFTWARE
  WoodwardBias : Inport
  Bus Creator : BusCreator  Inputs=4
  Bus Selector5 : BusSelector  OutputSignals=gen1_GOV_bias,gen1_AVR_bias
  Constant3 : Constant  Value=0
  Constant4 : Constant  Value=0
  Divide : Product  Inputs=*/
  Divide1 : Product  Inputs=*/
  Gen1 Ref AVR : Constant  Value=1.00
  Gen1 Ref GOV : Constant  Value=1.00
  Lowpass Filter : Subsystem  DialogController=fdesignblkfcn  DialogControllerArgs=DataTag6  InitFcn=fdesignblkfcn(gcbh, {'InitFcn'});  mask(Lowpass Filter){}
      mask help: Design a lowpass filter
      settings: CopyFcn=fdesignblkfcn(gcbh, {'CopyFcn'});
      mask Help: helpview(mapfilelocation('dsp'), 'dsplowpassfilter');
      mask Display: disp('Lowpass')
  Lowpass Filter1 : Subsystem  DialogController=fdesignblkfcn  DialogControllerArgs=DataTag8  InitFcn=fdesignblkfcn(gcbh, {'InitFcn'});  mask(Lowpass Filter){}
      mask help: Design a lowpass filter
      settings: CopyFcn=fdesignblkfcn(gcbh, {'CopyFcn'});
      mask Help: helpview(mapfilelocation('dsp'), 'dsplowpassfilter');
      mask Display: disp('Lowpass')
  ScalingBias : Constant  Value=20
  SimulatedBiasValues : Constant  Value=0
  Sum : Sum  Inputs=|+-
  Sum1 : Sum  Inputs=|+-
  Switch : Switch  Threshold=0.5
  Switch1 : Switch  Threshold=0.5
  bias_enable_for_woodward_ctrl : Constant
  Gen1 Gov and AVR : Outport
  wires:
  ScalingBias/1 -> Divide/2, Divide1/2
  Divide/1 -> Sum/1
  Divide1/1 -> Sum1/1
  Constant3/1 -> Sum/2
  Constant4/1 -> Sum1/2
  Sum/1 -> Lowpass Filter/1(In)
  Switch/1 -> Bus Creator/3  "Gen1 Gov"
  Switch1/1 -> Bus Creator/4  "Gen1 AVR"
  Sum1/1 -> Lowpass Filter1/1(In)
  SimulatedBiasValues/1 -> Switch/3, Switch1/3
  bias_enable_for_woodward_ctrl/1 -> Switch1/2, Switch/2
  Lowpass Filter/1(Out) -> Switch/1
  Lowpass Filter1/1(Out) -> Switch1/1
  Gen1 Ref AVR/1 -> Bus Creator/2  "Gen1 Ref AVR"
  Gen1 Ref GOV/1 -> Bus Creator/1  "Gen1 Ref GOV"
  Bus Creator/1 -> Gen1 Gov and AVR/1
  WoodwardBias/1 -> Bus Selector5/1
  Bus Selector5/1 -> Divide/1  "<gen1_GOV_bias>"
  Bus Selector5/2 -> Divide1/1  "<gen1_AVR_bias>"

== system BANSHEE/SS_PV_BESS/EPC/Controller Mapping/6-pulse RTE PWM generator (with deadtime) ==
  BL4 : Logic  Operator=NOT  Inputs=1
  Constant : Constant  Value=Internal_Phase
  "DeatTime [us] " : Constant  Value=Tdead
  Discrete Triangular-Waveform Generator : Subsystem  mask(Discrete Triangular-Waveform  Generator){Freq=Fc, Vpeak=1, Ts=Ts}
      mask prompts: Freq "Frequency (Hz):"; Vpeak "Peak value:"; Ts "Sample time:"
      mask init:
      | NumberStepsRounded=round(1/Freq/Ts);
      | % Selection of an even number of steps
      | if mod(NumberStepsRounded,2)==0
      |    NumberSteps=NumberStepsRounded;
      | else
      |    NumberSteps=NumberStepsRounded+1;
      | end
      | Freq_used=1/(NumberSteps*Ts);
  Gain : Gain  Gain=2*pi*Freq  SaturateOnIntegerOverflow=on  OutDataTypeStr=Inherit: Same as input  ParamDataTypeStr=Inherit: Same as input
  Gain2 : Gain  Gain=pi/180  SaturateOnIntegerOverflow=on  OutDataTypeStr=Inherit: Same as input  ParamDataTypeStr=Inherit: Same as input
  Mux : Mux  Inputs=2
  Mux2 : Mux  Inputs=2
  Product : Product  SaturateOnIntegerOverflow=on  InputSameDT=on  OutDataTypeStr=Inherit: Same as first input
  RTE Delay1 : rteventslib/Discrete/RTE Delay  IncMode=Enabled  DecMode=Disabled  IC=Low  BufferSize=2  MaxNbEvents=1
  RTE Logical Operator1 : rteventslib/Math Operations/RTE Logical Operator  LogicalOperator=AND  NbrInput=2  NbrMaxEvents=1
  RTE Logical Operator2 : rteventslib/Math Operations/RTE Logical Operator  LogicalOperator=NOR  NbrInput=2  NbrMaxEvents=1
  RTE Relational  Operator : rteventslib/Math Operations/RTE Relational Operator  RelationalOperator=<  NumberMaxEvents=1  SampleTime=Ts
  Relational Operator : RelationalOperator  InputSameDT=on
  Select1A : Selector  InputPortWidth=6  IndexOptions=Index vector (dialog)  Indices=Select1_Elements  OutputSizes=1
  Select1A2 : Selector  InputPortWidth=1  IndexOptions=Index vector (dialog)  Indices=[1 1 1]  OutputSizes=1
  Select1A3 : Selector  InputPortWidth=1  IndexOptions=Index vector (dialog)  Indices=[1 1 1]  OutputSizes=1
  Select1A4 : Selector  InputPortWidth=6  IndexOptions=Index vector (dialog)  Indices=Select1_Elements  OutputSizes=1
  Sum : Sum  Inputs=+++  SaturateOnIntegerOverflow=on  InputSameDT=on  OutDataTypeStr=Inherit: Same as first input
  Terminator1 : Terminator
  Trigonometric Function : Trigonometry
  m3 : Constant  Value=Phase
  m4 : Constant  Value=mIndex
  t : DigitalClock  SampleTime=Ts
  RTE : Outport
  SPS : Outport  Port=2
  wires:
  Select1A4/1 -> RTE/1
  Relational Operator/1 -> Mux/1, BL4/1
  t/1 -> Gain/1
  Gain/1 -> Sum/1
  Gain2/1 -> Sum/2
  m3/1 -> Gain2/1
  Constant/1 -> Sum/3
  m4/1 -> Product/1
  Sum/1 -> Trigonometric Function/1
  Trigonometric Function/1 -> Product/2
  Product/1 -> Relational Operator/1, RTE Relational  Operator/1
  Discrete Triangular-Waveform Generator/2(Freq_used) -> Terminator1/1
  BL4/1 -> Mux/2
  Mux/1 -> Select1A/1
  Discrete Triangular-Waveform Generator/1(Triangle) -> Select1A2/1
  Select1A/1 -> SPS/1
  RTE Logical Operator2/1 -> Mux2/2
  RTE Logical Operator1/1 -> Mux2/1
  RTE Delay1/1 -> RTE Logical Operator1/2, RTE Logical Operator2/2
  "DeatTime [us] "/1 -> Select1A3/1
  RTE Relational  Operator/1 -> RTE Logical Operator2/1, RTE Logical Operator1/1, RTE Delay1/1
  Select1A2/1 -> Relational Operator/2, RTE Relational  Operator/2
  Select1A3/1 -> RTE Delay1/2
  Mux2/1 -> Select1A4/1

== system BANSHEE/SS_PV_BESS/EPC/Controller Mapping/All Open ==
  note: This block wiill work for an 8 pulse Sim Power Systems
      | switching model where all are zeros is ok. It will not work
      | with an RTE block because of how the power electronics model.
  Bus Creator1 : BusCreator  Inputs=8
  GD1_8 : Constant  Value=0
  Pulses8 : Outport
  wires:
  GD1_8/1 -> Bus Creator1/1, Bus Creator1/2, Bus Creator1/3, Bus Creator1/4, Bus Creator1/5, Bus Creator1/6, Bus Creator1/7, Bus Creator1/8
  Bus Creator1/1 -> Pulses8/1

== system BANSHEE/SS_PV_BESS/EPC/Controller Mapping/BESS Signal Mapping ==
  In1 : Inport
  Bus Creator : BusCreator  Inputs=6
  Bus Creator1 : BusCreator  Inputs=6
  Constant : Constant
  Demux : Demux  Outputs=6
  Demux1 : Demux  Outputs=6
  RTE Conversion : rteventslib/Signal Attributes/RTE Conversion  inputdatatype=Double  outputdatatype=RTE Boolean  compensation=Enabled  nbMaxEvents=4  sampleTime=Ts
  RTE Conversion1 : rteventslib/Signal Attributes/RTE Conversion  inputdatatype=RTE Boolean  outputdatatype=Double  compensation=Enabled  nbMaxEvents=4  sampleTime=Ts
  RTE Logical Operator : rteventslib/Math Operations/RTE Logical Operator  LogicalOperator=NOR  NbrInput=6  NbrMaxEvents=4
  RTE Switch : rteventslib/Signal Routing/RTE Switch  switchType=u2 = Double; u1 u3 = RTE Boolean  criteria=u2 >= Threshold  threshold=0.5  interpolate=on  nbMaxEvents=4
  RTE Switch1 : rteventslib/Signal Routing/RTE Switch  switchType=u2 = Double; u1 u3 = RTE Boolean  criteria=u2 >= Threshold  threshold=0.5  interpolate=on  nbMaxEvents=4
  RTE Switch2 : rteventslib/Signal Routing/RTE Switch  switchType=u2 = Double; u1 u3 = RTE Boolean  criteria=u2 >= Threshold  threshold=0.5  interpolate=on  nbMaxEvents=4
  TSD_RTE : Outport
  TSD_RTE_v2 : Outport  Port=2
  wires:
  Bus Creator1/1 -> TSD_RTE_v2/1
  Demux1/6 -> Bus Creator1/6  "Phase 3 Bottom"
  Demux1/5 -> Bus Creator1/5  "Phase 3 Top"
  Demux1/4 -> Bus Creator1/4  "Phase 2 Bottom"
  Demux1/3 -> Bus Creator1/3  "Phase 2 Top"
  Demux1/2 -> Bus Creator1/2  "Phase 1 Bottom"
  Demux1/1 -> Bus Creator1/1  "Phase 1 Top"
  In1/1 -> Demux/1, Demux1/1
  RTE Switch2/1 -> Bus Creator/6
  RTE Switch1/1 -> Bus Creator/4
  RTE Switch/1 -> Bus Creator/2
  Demux/1 -> RTE Logical Operator/1, Bus Creator/1  "Phase 1 Bot Switch"
  Demux/2 -> RTE Logical Operator/2, RTE Switch/3  "Phase 1 Top Switch"
  Demux/3 -> Bus Creator/3, RTE Logical Operator/3  "Phase 2 Bot Switch"
  Demux/4 -> RTE Logical Operator/4, RTE Switch1/3  "Phase 2 Top Switch"
  Demux/5 -> RTE Logical Operator/5, Bus Creator/5  "Phase 3 Bot Switch"
  Demux/6 -> RTE Logical Operator/6, RTE Switch2/3  "Phase 3 Top Switch"
  Bus Creator/1 -> TSD_RTE/1  "TSD_RTE"
  RTE Logical Operator/1 -> RTE Conversion1/1
  Constant/1 -> RTE Conversion/1
  RTE Conversion/1 -> RTE Switch/1, RTE Switch1/1, RTE Switch2/1
  RTE Conversion1/1 -> RTE Switch2/2, RTE Switch/2, RTE Switch1/2

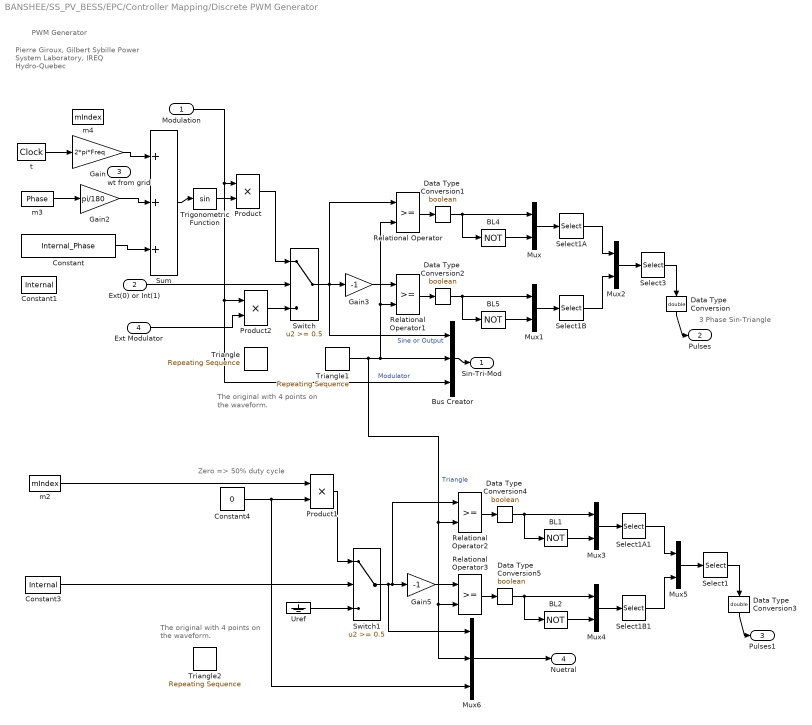
== system BANSHEE/SS_PV_BESS/EPC/Controller Mapping/Discrete PWM Generator ==
  note: Pierre Giroux, Gilbert Sybille
      | Power System Laboratory, IREQ
      | Hydro-Quebec
  note: PWM Generator
  note: 3 Phase
      | Sin-Triangle
  note: Zero => 50% duty cycle
  note: The original with 4
      | points on the waveform.
  note: The original with 4
      | points on the waveform.
  Modulation : Inport
  Ext(0) or Int(1) : Inport  Port=2
  wt from grid : Inport  Port=3
  Ext Modulator : Inport  Port=4
  BL{1..2,4..5} (4 alike) : Logic  Operator=NOT  Inputs=1  SampleTime=Ts
  Bus Creator : BusCreator  Inputs=3
  Constant : Constant  Value=Internal_Phase  SampleTime=Ts
  Constant1 : Constant  Value=Internal  SampleTime=Ts
  Constant3 : Constant  Value=Internal  SampleTime=Ts
  Constant4 : Constant  Value=0
  Data Type  Conversion : DataTypeConversion  OutDataTypeStr=double  SampleTime=Ts  SaturateOnIntegerOverflow=on  RndMeth=Zero
  Data Type  Conversion{1..2,4..5} (4 alike) : DataTypeConversion  OutDataTypeStr=boolean  SampleTime=Ts  SaturateOnIntegerOverflow=on  RndMeth=Zero
  Data Type  Conversion3 : DataTypeConversion  OutDataTypeStr=double  SampleTime=Ts  SaturateOnIntegerOverflow=on  RndMeth=Zero
  Gain : Gain  Gain=2*pi*Freq  SaturateOnIntegerOverflow=on  OutDataTypeStr=Inherit: Same as input  ParamDataTypeStr=Inherit: Same as input
  Gain2 : Gain  Gain=pi/180  SaturateOnIntegerOverflow=on  OutDataTypeStr=Inherit: Same as input  ParamDataTypeStr=Inherit: Same as input
  Gain3 : Gain  Gain=-1  SampleTime=Ts  SaturateOnIntegerOverflow=on  OutDataTypeStr=Inherit: Same as input  ParamDataTypeStr=Inherit: Same as input
  Gain5 : Gain  Gain=-1  SampleTime=Ts  SaturateOnIntegerOverflow=on  OutDataTypeStr=Inherit: Same as input  ParamDataTypeStr=Inherit: Same as input
  Mux{,1..5} (6 alike) : Mux  Inputs=2
  Mux6 : Mux  Inputs=3
  Product : Product  SampleTime=Ts  SaturateOnIntegerOverflow=on  InputSameDT=on  OutDataTypeStr=Inherit: Same as first input
  Product1 : Product  SampleTime=Ts  SaturateOnIntegerOverflow=on  InputSameDT=on  OutDataTypeStr=Inherit: Same as first input
  Product2 : Product  SampleTime=Ts  SaturateOnIntegerOverflow=on  InputSameDT=on  OutDataTypeStr=Inherit: Same as first input
  Relational Operator{,1..3} (4 alike) : RelationalOperator  SampleTime=Ts  InputSameDT=on
  Select1 : Selector  InputPortWidth=Select3_PortWidth  IndexOptions=Index vector (dialog)  Indices=Select3_Elements  OutputSizes=1
  Select1A : Selector  InputPortWidth=Select1_PortWidth  IndexOptions=Index vector (dialog)  Indices=Select1_Elements  OutputSizes=1
  Select1A1 : Selector  InputPortWidth=Select1_PortWidth  IndexOptions=Index vector (dialog)  Indices=Select1_Elements  OutputSizes=1
  Select1B : Selector  InputPortWidth=Select1_PortWidth  IndexOptions=Index vector (dialog)  Indices=Select1_Elements  OutputSizes=1
  Select1B1 : Selector  InputPortWidth=Select1_PortWidth  IndexOptions=Index vector (dialog)  Indices=Select1_Elements  OutputSizes=1
  Select3 : Selector  InputPortWidth=Select3_PortWidth  IndexOptions=Index vector (dialog)  Indices=Select3_Elements  OutputSizes=1
  Sum : Sum  Inputs=+++  SampleTime=Ts  SaturateOnIntegerOverflow=on  InputSameDT=on  OutDataTypeStr=Inherit: Same as first input
  Switch : Switch  Threshold=0.5  SampleTime=Ts  SaturateOnIntegerOverflow=on  InputSameDT=on
  Switch1 : Switch  Threshold=0.5  SampleTime=Ts  SaturateOnIntegerOverflow=on  InputSameDT=on
  Triangle : simulink/Sources/Repeating Sequence  rep_seq_t=[0 1/Fc/4 3/Fc/4 1/Fc]  rep_seq_y=[0 -1 1 0]
  Triangle1 : simulink/Sources/Repeating Sequence  rep_seq_t=[0 1/Fc/2 1/Fc]  rep_seq_y=[-1 1 -1]
  Triangle2 : simulink/Sources/Repeating Sequence  rep_seq_t=[0 1/Fc/4 3/Fc/4 1/Fc]  rep_seq_y=[0 -1 1 0]
  Trigonometric Function : Trigonometry  SampleTime=Ts
  Uref : Ground
  m2 : Constant  Value=mIndex  SampleTime=Ts
  m3 : Constant  Value=Phase  SampleTime=Ts
  m4 : Constant  Value=mIndex  SampleTime=Ts
  t : DigitalClock  SampleTime=Ts
  Sin-Tri-Mod : Outport  SampleTime=Ts
  Pulses : Outport  Port=2  SampleTime=Ts
  Pulses1 : Outport  Port=3  SampleTime=Ts
  Nuetral : Outport  Port=4  SampleTime=Ts
  wires:
  Switch/1 -> Relational Operator/1, Gain3/1, Bus Creator/1  "Sine or Output"
  Mux2/1 -> Select3/1
  Select1B/1 -> Mux2/2
  Select1A/1 -> Mux2/1
  Mux1/1 -> Select1B/1
  Mux/1 -> Select1A/1
  BL5/1 -> Mux1/2
  BL4/1 -> Mux/2
  Gain3/1 -> Relational Operator1/1
  Product/1 -> Switch/1
  Trigonometric Function/1 -> Product/2
  Sum/1 -> Trigonometric Function/1
  m3/1 -> Gain2/1
  t/1 -> Gain/1
  Select3/1 -> Data Type  Conversion/1
  Data Type  Conversion/1 -> Pulses/1
  Relational Operator/1 -> Data Type  Conversion1/1
  Data Type  Conversion1/1 -> BL4/1, Mux/1
  Relational Operator1/1 -> Data Type  Conversion2/1
  Data Type  Conversion2/1 -> BL5/1, Mux1/1
  Bus Creator/1 -> Sin-Tri-Mod/1
  Triangle1/1 -> Bus Creator/2, Relational Operator1/2, Relational Operator/2, Relational Operator3/2, Mux6/2, Relational Operator2/2  "Triangle"
  Switch1/1 -> Relational Operator2/1, Gain5/1, Mux6/1
  Mux5/1 -> Select1/1
  Select1B1/1 -> Mux5/2
  Select1A1/1 -> Mux5/1
  Mux4/1 -> Select1B1/1
  Mux3/1 -> Select1A1/1
  BL2/1 -> Mux4/2
  BL1/1 -> Mux3/2
  Gain5/1 -> Relational Operator3/1
  Product1/1 -> Switch1/1
  m2/1 -> Product1/1
  Select1/1 -> Data Type  Conversion3/1
  Data Type  Conversion3/1 -> Pulses1/1
  Relational Operator2/1 -> Data Type  Conversion4/1
  Data Type  Conversion4/1 -> BL1/1, Mux3/1
  Relational Operator3/1 -> Data Type  Conversion5/1
  Data Type  Conversion5/1 -> BL2/1, Mux4/1
  Constant4/1 -> Product1/2, Mux6/3
  Mux6/1 -> Nuetral/1
  Product2/1 -> Switch/3
  Constant3/1 -> Switch1/2
  Uref/1 -> Switch1/3
  Ext(0) or Int(1)/1 -> Switch/2
  Modulation/1 -> Bus Creator/3, Product2/1, Product/1  "Modulator"
  Ext Modulator/1 -> Product2/2
  Constant/1 -> Sum/3
  Gain2/1 -> Sum/2
  Gain/1 -> Sum/1

== system BANSHEE/SS_PV_BESS/EPC/Controller Mapping/EPC Inverter Controller Outputs ==
  note: These PWM IN Signals will be used.
      | PWM 1 and 2 are Bot and Top
      | PWM 3 and 4 are Bot and Top
      | PWM 5 and 6 are Bot and Top
  note: When using TSD set the DOUT type config to 0
      | When using PWM set the DOUT type config to 1
  note: It was at 1 for PWM, but it seems that
      | it is better to use the event detector conversion
      | block with TSD instead.
  Console Input : Inport
  Bus Creator1 : BusCreator  Inputs=3
  Bus Creator2 : BusCreator  Inputs=2
  Bus Selector1 : BusSelector  OutputSignals=00-03,04-07  OutputAsBus=on
  Bus Selector2 : BusSelector  OutputSignals=08-11,12-15  OutputAsBus=on
  Bus Selector6 : BusSelector  OutputSignals=16 DOUT GR3,16 TSDOUT GR3,16 PWMOUT GR3
  DIO - Gr4 : Subsystem
  DOUT type config : Subsystem
  GR1 B AIN (CH00-15) : Subsystem
  OpCtrl OP5142EX2 : rtio_opalrt_op5142ex1/OpCtrl OP5142EX1  CtrlName='OP5142EX2 Ctrl'  boardid=2  BitstreamFilename=OP5142_1-EX-0000-2_3_4_54-16AIO_48AO_16DIO_16selDIO_CD-FF-01.bin  numconfig=-1  mode=Slave  externalClock=off  decimRtsi=0  calibIO=off  SampleTime=0  loadinport=-1
  PWM IO - Gr4 : Subsystem
  TSDIO - Gr4 : Subsystem
  Error : Outport
  IDs : Outport  Port=2
  PWM : Outport  Port=3
  Digital Inputs : Outport  Port=4
  PWM_RTE : Outport  Port=5
  BESS_TSD_RTE : Outport  Port=6
  PV_TSD_RTE : Outport  Port=7
  wires:
  TSDIO - Gr4/3(PV_TSDin_RTE) -> PV_TSD_RTE/1
  OpCtrl OP5142EX2/1 -> Error/1
  OpCtrl OP5142EX2/2 -> IDs/1
  PWM IO - Gr4/1(PWMIn) -> Bus Creator1/3, PWM/1  "PWMIN"
  TSDIO - Gr4/1(TSDin) -> Bus Creator1/2  "TSDIN"
  DIO - Gr4/1(DIn) -> Bus Creator1/1  "DIN"
  Bus Creator1/1 -> Digital Inputs/1
  Console Input/1 -> Bus Selector6/1
  Bus Selector6/2 -> TSDIO - Gr4/1(TSDout)  "<16 TSDOUT GR3>"
  Bus Selector6/3 -> PWM IO - Gr4/1(PWMOut)  "<16 PWMOUT GR3>"
  Bus Selector6/1 -> Bus Selector1/1, Bus Selector2/1  "<16 DOUT GR3>"
  Bus Selector1/1 -> Bus Creator2/1  "DI_CH00-07"
  Bus Selector2/1 -> Bus Creator2/2  "DI_CH08-15"
  Bus Creator2/1 -> DIO - Gr4/1(Dout)
  PWM IO - Gr4/2(PWMIn_RTE) -> PWM_RTE/1
  TSDIO - Gr4/2(BESS_TSDin_RTE) -> BESS_TSD_RTE/1
